simulink model "toplivo2017a"  (R2017a)
settings: Solver=ode1  StartTime=0.0  StopTime=inf  FixedStep=0.01  RelTol=1e-3  EnableMultiTasking=on
undefined symbols (not defined in the file or in its folder): components_Component_PID_instance_3_cD_Max, components_Component_PID_instance_3_cD_Min, components_Component_PID_instance_3_cI_Max, components_Component_PID_instance_3_cI_Min, components_Component_PID_instance_3_cP_Max, components_Component_PID_instance_3_cP_Min
libraries: SIPLib x1
settings Model: Creator=Stud_58  LastModifiedBy=Пользователь
settings DataIOCC: LimitDataPoints=on  SaveFormat=Array
settings OptimizationCC: ExpressionDepthLimit=2147483647  LifeSpan=inf
settings DebuggingCC: UnderspecifiedInitializationDetection=Classic  MergeDetectMultiDrivingBlocksExec=none  SolverPrmCheckMsg=warning  FcnCallInpInsideContextMsg=warning  StateNameClashWarn=warning  SFUnexpectedBacktrackingDiag=warning  SFNoUnconditionalDefaultTransitionDiag=warning  SFExecutionAtInitializationDiag=none
settings HardwareCC: ProdBitPerPointer=32  ProdBitPerSizeT=32  ProdBitPerPtrDiffT=32  ProdLargestAtomicFloat=None  ProdIntDivRoundTo=Undefined  ProdEndianess=Unspecified  ProdWordSize=32  ProdHWDeviceType=32-bit Generic
settings ModelReferenceCC: PropagateSignalLabelsOutOfModel=off
settings GRTTargetCC: TargetLangStandard=C89/C90 (ANSI)  GeneratePreprocessorConditionals=Disable all  CombineOutputUpdateFcns=off  GRTInterface=on
settings ConfigComp: CovMetricSettings=dw  CovHtmlReporting=on  CovSaveCumulativeToWorkspaceVar=on  CovSaveSingleToWorkspaceVar=on  CovExternalEMLEnable=off

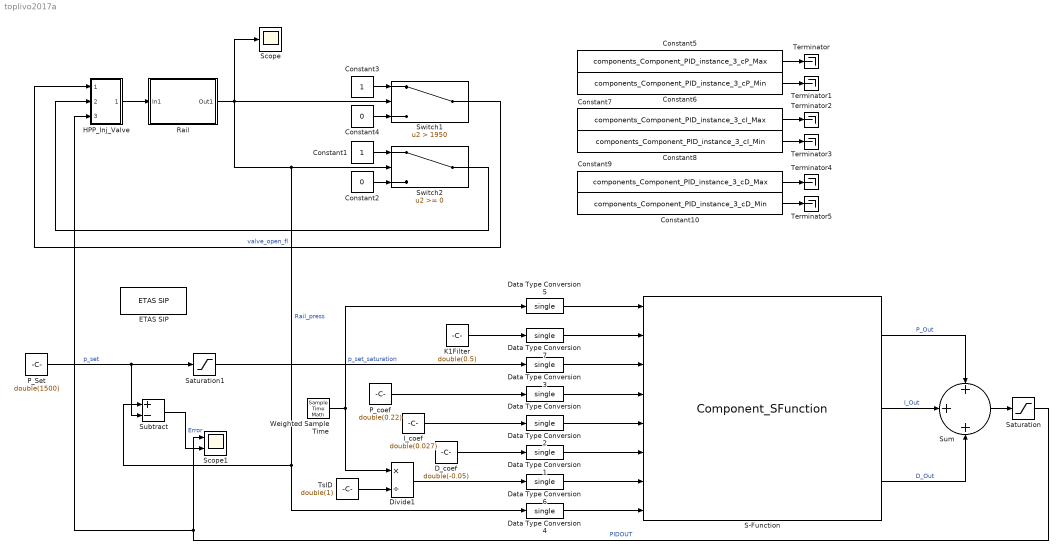
== system toplivo2017a ==
  Constant1 : Constant
  Constant10 : Constant  Value=components_Component_PID_instance_3_cD_Min
  Constant2 : Constant  Value=0
  Constant3 : Constant
  Constant4 : Constant  Value=0
  Constant5 : Constant  Value=components_Component_PID_instance_3_cP_Max
  Constant6 : Constant  Value=components_Component_PID_instance_3_cP_Min
  Constant7 : Constant  Value=components_Component_PID_instance_3_cI_Max
  Constant8 : Constant  Value=components_Component_PID_instance_3_cI_Min
  Constant9 : Constant  Value=components_Component_PID_instance_3_cD_Max
  D_coef : Constant  Value=double(-0.05)
  Data Type Conversion{,1..7} (8 alike) : DataTypeConversion  OutDataTypeStr=single
  Divide1 : Product  Inputs=*/
  ETAS SIP : SIPLib/ETAS SIP
  HPP_Inj_Valve : Subsystem
  I_coef : Constant  Value=double(0.027)
  "K1Filter " : Constant  Value=double(0.5)
  "P_Set " : Constant  Value=double(1500)
  P_coef : Constant  Value=double(0.22)
  Rail : Subsystem
  S-Function : S-Function  InitFcn=clear Component_SFunction  FunctionName=Component_SFunction  Parameters=components_Component_PID_instance_cP_Max components_Component_PID_instance_cP_Min components_Component_PID_instance_cI_Max components_Component_PID_instance_cD_Max components_Component_PID_instance_cD_Min components_Component_PID_instance_cI_Min components_Component_RunningAverage_instance_c1 components_Component_FilterBy_instance_K2 components_Component_PID_instance_3_cP_Max components_Component_PID_instance_3_cP_Min components_Component_PID_instance_3_cI_Max components_Component_PID_instance_3_cD_Max components_Component_PID_instance_3_cD_Min components_Component_PID_instance_3_cI_Min  SFunctionDeploymentMode=off  EnableBusSupport=off
      mask Display:
      | disp('Component_SFunction')
      | port_label('output',1,'components.InpOut.P_Out')
      | port_label('output',2,'components.InpOut.I_Out')
      | port_label('output',3,'components.InpOut.D_Out')
      | port_label('input',1,'components.Filter.TsFilter')
      | port_label('input',2,'components.Filter.K1')
      | port_label('input',3,'components.PID.PressSet')
      | port_label('input',4,'components.PID.qP')
      | port_label('input',5,'components.PID.qI')
      | port_label('input',6,'components.PID.qD')
      | port_label('input',7,'components.PID.TsPID')
      | port_label('input',8,'components.InpOut.Input')
  Saturation : Saturate  UpperLimit=100  LowerLimit=0
  Saturation1 : Saturate  UpperLimit=2000  LowerLimit=-0.0
  Scope : Scope
  Scope1 : Scope  NumInputPorts=2
  Subtract : Sum  Inputs=+-
  Sum : Sum  Inputs=+++
  Switch1 : Switch  Criteria=u2 > Threshold  Threshold=1950
  Switch2 : Switch
  Terminator{,1..5} (6 alike) : Terminator
  TsID : Constant  Value=double(1)
  Weighted Sample Time : SampleTimeMath  TsampMathOp=Ts Only
  wires:
  Switch1/1 -> HPP_Inj_Valve/1(In1)  "valve_open_fl"
  Rail/1(Out1) -> Subtract/1, Data Type Conversion4/1, Switch2/2, Switch1/2, Scope/1  "Rail_press"
  Constant3/1 -> Switch1/1
  Constant4/1 -> Switch1/3
  "P_Set "/1 -> Subtract/2, Saturation1/1  "p_set"
  HPP_Inj_Valve/1(Out1) -> Rail/1(In1)
  Constant2/1 -> Switch2/3
  Constant1/1 -> Switch2/1
  Switch2/1 -> HPP_Inj_Valve/2(In2)
  Saturation/1 -> Scope1/1, HPP_Inj_Valve/3(In3)  "PIDOUT"
  P_coef/1 -> Data Type Conversion/1
  Data Type Conversion/1 -> S-Function/4
  I_coef/1 -> Data Type Conversion2/1
  Data Type Conversion2/1 -> S-Function/5
  D_coef/1 -> Data Type Conversion1/1
  Data Type Conversion1/1 -> S-Function/6
  Saturation1/1 -> Data Type Conversion3/1  "p_set_saturation"
  Data Type Conversion3/1 -> S-Function/3
  Data Type Conversion4/1 -> S-Function/8
  Weighted Sample Time/1 -> Data Type Conversion5/1, Divide1/1
  Data Type Conversion5/1 -> S-Function/1
  Sum/1 -> Saturation/1
  Subtract/1 -> Scope1/2  "Error"
  TsID/1 -> Divide1/2
  Divide1/1 -> Data Type Conversion6/1
  Data Type Conversion6/1 -> S-Function/7
  "K1Filter "/1 -> Data Type Conversion7/1
  Data Type Conversion7/1 -> S-Function/2
  S-Function/2 -> Sum/2  "I_Out"
  S-Function/1 -> Sum/1  "P_Out"
  S-Function/3 -> Sum/3  "D_Out"
  Constant6/1 -> Terminator1/1
  Constant5/1 -> Terminator/1
  Constant7/1 -> Terminator2/1
  Constant8/1 -> Terminator3/1
  Constant9/1 -> Terminator4/1
  Constant10/1 -> Terminator5/1

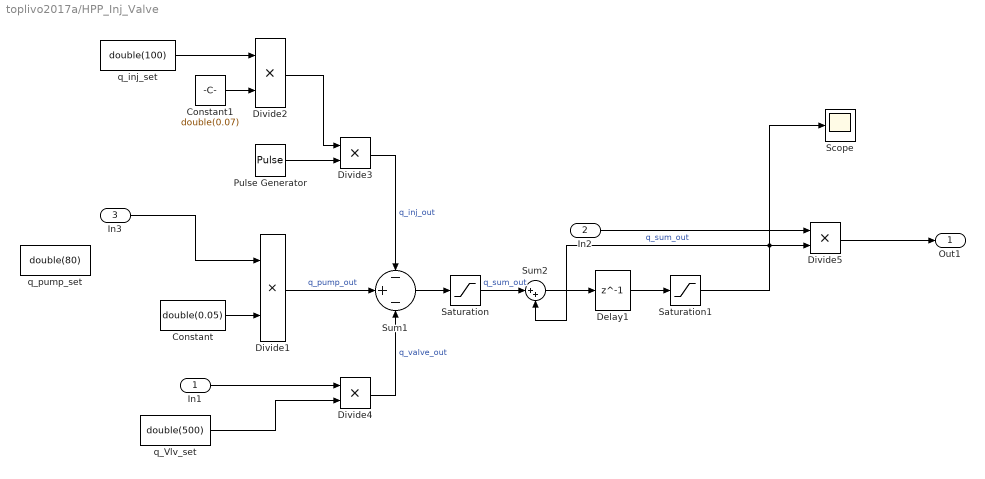
== system toplivo2017a/HPP_Inj_Valve ==
  In1 : Inport
  In2 : Inport  Port=2
  In3 : Inport  Port=3
  Constant : Constant  Value=double(0.05)
  Constant1 : Constant  Value=double(0.07)
  Delay1 : Delay  DelayLength=1
  Divide{1..5} (5 alike) : Product  Inputs=**
  Pulse Generator : DiscretePulseGenerator  PulseType=Time based  Amplitude=0.4  Period=0.3  PulseWidth=10
  Saturation : Saturate  UpperLimit=100  LowerLimit=-1000
  Saturation1 : Saturate  UpperLimit=inf  LowerLimit=0
  Scope : Scope
  Sum1 : Sum  Inputs=-+-
  Sum2 : Sum  Inputs=|++
  q_Vlv_set : Constant  Value=double(500)
  q_inj_set : Constant  Value=double(100)
  "q_pump_set " : Constant  Value=double(80)
  Out1 : Outport
  wires:
  Constant/1 -> Divide1/2
  q_inj_set/1 -> Divide2/1
  Constant1/1 -> Divide2/2
  Sum1/1 -> Saturation/1
  Divide3/1 -> Sum1/1  "q_inj_out"
  Sum2/1 -> Delay1/1
  Pulse Generator/1 -> Divide3/2
  Delay1/1 -> Saturation1/1
  Divide1/1 -> Sum1/2  "q_pump_out"
  Divide2/1 -> Divide3/1
  q_Vlv_set/1 -> Divide4/2
  In1/1 -> Divide4/1
  Divide4/1 -> Sum1/3  "q_valve_out"
  Divide5/1 -> Out1/1
  In2/1 -> Divide5/1
  Saturation/1 -> Sum2/1  "q_sum_out"
  Saturation1/1 -> Sum2/2, Scope/1, Divide5/2  "q_sum_out"
  In3/1 -> Divide1/1

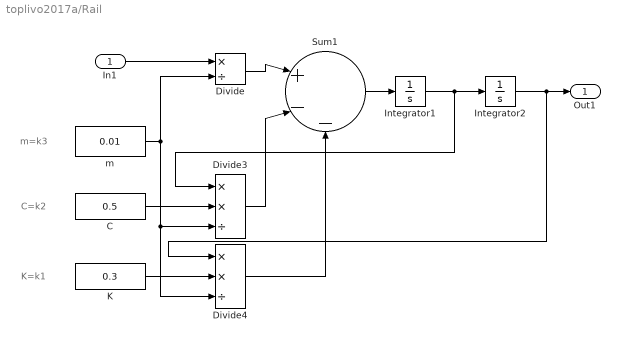
== system toplivo2017a/Rail ==
  note: K=k1
  note: C=k2
  note: m=k3
  In1 : Inport
  C : Constant  Value=0.5
  Divide : Product  Inputs=*/
  Divide3 : Product  Inputs=**/
  Divide4 : Product  Inputs=**/
  Integrator1 : Integrator
  Integrator2 : Integrator
  K : Constant  Value=0.3
  Sum1 : Sum  Inputs=|+--
  m : Constant  Value=0.01
  Out1 : Outport
  wires:
  In1/1 -> Divide/1
  Integrator2/1 -> Divide4/1, Out1/1
  Divide/1 -> Sum1/1
  Sum1/1 -> Integrator1/1
  Integrator1/1 -> Divide3/1, Integrator2/1
  m/1 -> Divide4/3, Divide3/3, Divide/2
  C/1 -> Divide3/2
  K/1 -> Divide4/2
  Divide4/1 -> Sum1/3
  Divide3/1 -> Sum1/2
